simulink model "limit_test_function"  (R2018b)
settings: Solver=FixedStepAuto  StartTime=0.0  StopTime=50  FixedStep=0.001  RelTol=1e-3
libraries: simulink x1
settings Model: Creator=Paweł Tymiński  LastModifiedBy=Paweł Tymiński

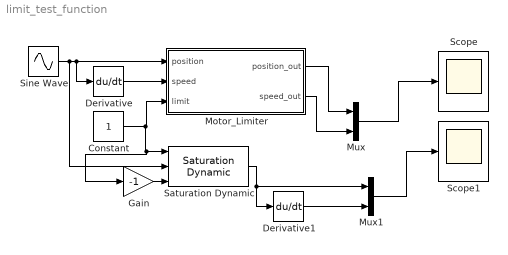
== system limit_test_function ==
  Constant : Constant
  Derivative : Derivative
  Derivative1 : Derivative
  Gain : Gain  Gain=-1
  Motor_Limiter : MATLAB Function  TreatAsAtomicUnit=on
  Mux : Mux  Inputs=2
  Mux1 : Mux  Inputs=2
  Saturation Dynamic : simulink/Discontinuities/Saturation Dynamic  OutMin=[]  OutMax=[]  OutDataTypeStr=Inherit: Same as second input  OutDataType=fixdt(1, 16)  OutScaling=2^-10  DoSatur=off
  Scope : Scope
  Scope1 : Scope
  Sine Wave : Sin  Amplitude=2  SampleTime=0
  wires:
  Sine Wave/1 -> Saturation Dynamic/2, Derivative/1, Motor_Limiter/1(position)
  Derivative/1 -> Motor_Limiter/2(speed)
  Constant/1 -> Gain/1, Saturation Dynamic/1, Motor_Limiter/3(limit)
  Saturation Dynamic/1 -> Mux1/1, Derivative1/1
  Derivative1/1 -> Mux1/2
  Mux1/1 -> Scope1/1
  Mux/1 -> Scope/1
  Motor_Limiter/1(position_out) -> Mux/1
  Motor_Limiter/2(speed_out) -> Mux/2
  Gain/1 -> Saturation Dynamic/3

== matlab function limit_test_function/Motor_Limiter ==
  data: position input; position_out output; speed input; speed_out output; limit input
function [position_out,speed_out] = fcn(position, speed, limit)
if abs(position)<limit        
    position_out=position;
    speed_out=speed;
else
    position_out=sign(position)*limit;   
    speed_out=0;
end
